simulink model "simulation"  (R2022b)
settings: Solver=FixedStepAuto  StartTime=0.0  StopTime=15  FixedStep=0.01  RelTol=1e-3
settings Model: Creator=lrf  LastModifiedBy=lrf

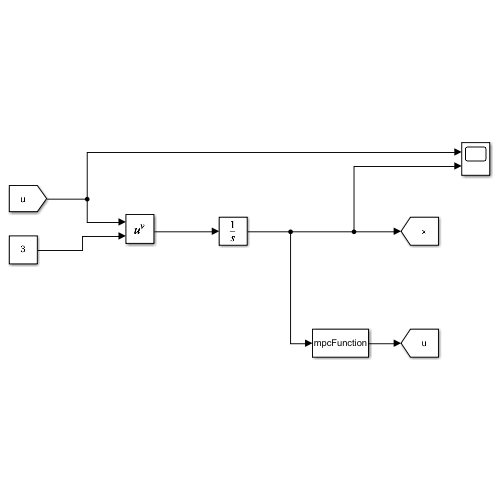
[thumbnail: Simulink's stored preview of the top-level diagram]
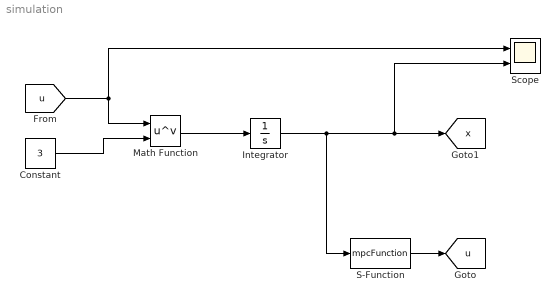
== system simulation ==
  Constant : Constant  Value=3
  Integrator : Integrator
  Math Function : Math  Operator=pow
  S-Function : S-Function  FunctionName=mpcFunction  SFunctionDeploymentMode=off  EnableBusSupport=off
  Scope : Scope  NumInputPorts=2
  tag scope: u=global, x=global
  wires:
  Integrator/1 -> S-Function/1, Scope/2, [x]
  Math Function/1 -> Integrator/1
  S-Function/1 -> [u]
  Constant/1 -> Math Function/2
  [u] -> Math Function/1, Scope/1
